simulink model "llc_ctrl_model"  (R2020a)
settings: Solver=ode45  StartTime=0.0  StopTime=1  RelTol=1e-3
undefined symbols (not defined in the file or in its folder): llc_ctrl_cfg_default
libraries: powerlib x19, commsynccomp2 x1
settings Model: Creator=huyan  LastModifiedBy=huyan

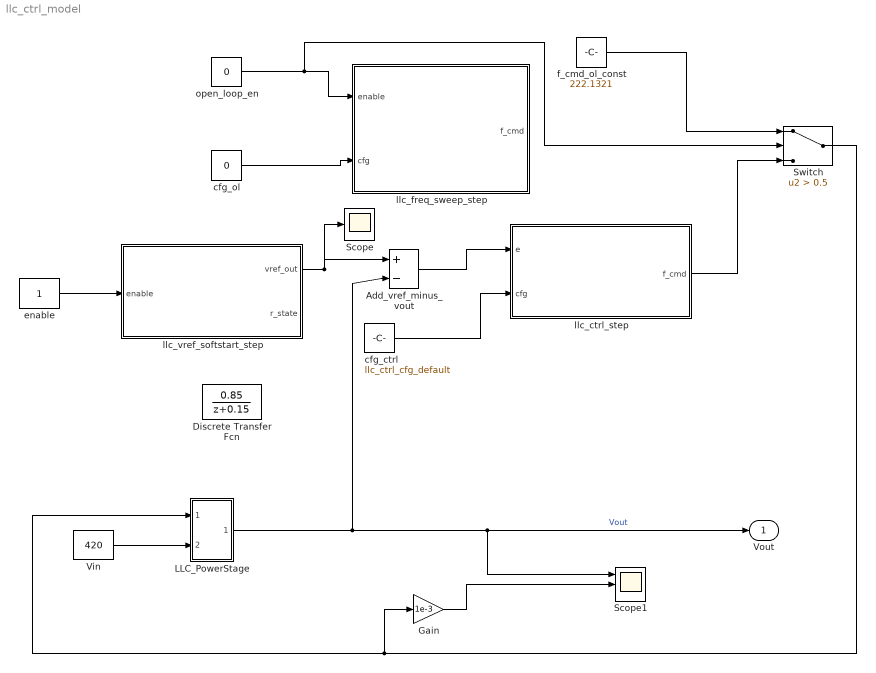
== system llc_ctrl_model ==
  Add_vref_minus_vout : Sum  Inputs=|+-
  Discrete Transfer Fcn : DiscreteTransferFcn  Numerator=0.85  Denominator=[1 0.15]  InitialStates=44  SampleTime=1e-4
  Gain : Gain  Gain=1e-3
  LLC_PowerStage : Subsystem
  Scope : Scope
  Scope1 : Scope  NumInputPorts=3
  Switch : Switch  Criteria=u2 > Threshold  Threshold=0.5
  Vin : Constant  Value=420  SampleTime=0.0001
  cfg_ctrl : Constant  Value=llc_ctrl_cfg_default  OutDataTypeStr=Bus: LLC_CTRL_CFG
  cfg_ol : Constant  Value=0  OutDataTypeStr=Bus: LLC_OL_CFG
  enable : Constant  SampleTime=0.0001
  f_cmd_ol_const : Constant  Value=222.1321
  llc_ctrl_step : MATLAB Function  TreatAsAtomicUnit=on  SystemSampleTime=1e-4
  "llc_freq_sweep_step " : MATLAB Function  TreatAsAtomicUnit=on
  llc_vref_softstart_step : MATLAB Function  TreatAsAtomicUnit=on  SystemSampleTime=1e-4
  open_loop_en : Constant  Value=0  OutDataTypeStr=double
  Vout : Outport
  wires:
  enable/1 -> llc_vref_softstart_step/1(enable)
  llc_vref_softstart_step/1(vref_out) -> Scope/1, Add_vref_minus_vout/1
  Add_vref_minus_vout/1 -> llc_ctrl_step/1(e)
  Vin/1 -> LLC_PowerStage/2(Vin)
  LLC_PowerStage/1(Vout) -> Add_vref_minus_vout/2, Vout/1, Scope1/1  "Vout"
  open_loop_en/1 -> "llc_freq_sweep_step "/1(enable), Switch/2
  cfg_ol/1 -> "llc_freq_sweep_step "/2(cfg)
  cfg_ctrl/1 -> llc_ctrl_step/2(cfg)
  Gain/1 -> Scope1/2
  f_cmd_ol_const/1 -> Switch/1
  llc_ctrl_step/1(f_cmd) -> Switch/3
  Switch/1 -> Gain/1, LLC_PowerStage/1(f_cmd)

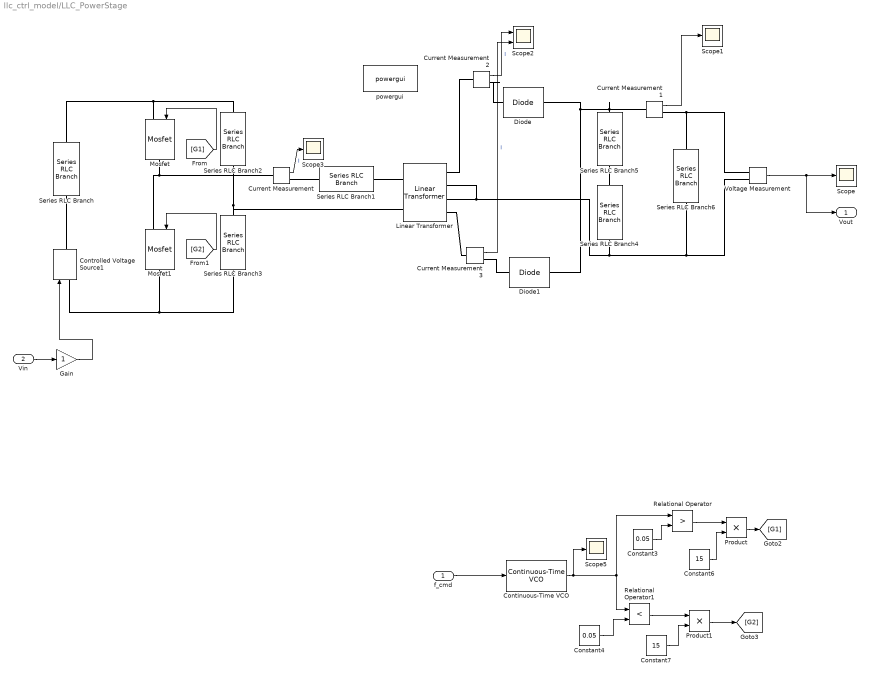
== system llc_ctrl_model/LLC_PowerStage ==
  f_cmd : Inport
  Vin : Inport  Port=2
  Constant3 : Constant  Value=0.05
  Constant4 : Constant  Value=0.05
  Constant6 : Constant  Value=15
  Constant7 : Constant  Value=15
  Continuous-Time VCO : commsynccomp2/Continuous-Time VCO  Ac=1  Fc=0  Kc=1  Ph=0
      settings: SourceProductBaseCode=CM
  Controlled Voltage Source1 : powerlib/Electrical Sources/Controlled Voltage Source  Initialize=on  Source_Type=AC  Amplitude=0  Phase=0  Frequency=0  Measurements=None
  Current Measurement{,1..3} (4 alike) : powerlib/Measurements/Current Measurement  PhasorSimulation=off  OutputType=Complex  PSBequivalent=0
  Diode : powerlib/Power Electronics/Diode  Ron=0.001  Lon=0  Vf=1.5  IC=0  UseSnubber=0  Rs=0.8  Cs=1e-9  Measurements=off
  Diode1 : powerlib/Power Electronics/Diode  Ron=0.001  Lon=0  Vf=1.5  IC=0  UseSnubber=0  Rs=0.8  Cs=1e-9  Measurements=off
  Gain : Gain
  Linear Transformer : powerlib/Elements/Linear Transformer  UNITS=SI  NominalPower=[ 3000 100000 ]  winding1=[300 0 0]  winding2=[63.1 0 0]  ThreeWindings=on  winding3=[63.1 0 0]  RmLm=[2.888e+08 0.000077]  Measurements=None  DataType=on
  Mosfet : powerlib/Power Electronics/Mosfet  Ron=0.1  Lon=0  Rd=0.01  Vfd=0  IC=0  Rs=1e5  Cs=inf  Measurements=off
  Mosfet1 : powerlib/Power Electronics/Mosfet  Ron=0.1  Lon=0  Rd=0.01  Vfd=0  IC=0  Rs=1e5  Cs=inf  Measurements=off
  Product : Product
  Product1 : Product
  Relational Operator : RelationalOperator  Operator=>  OutDataTypeStr=boolean  RndMeth=Simplest
  Relational Operator1 : RelationalOperator  Operator=<  OutDataTypeStr=boolean  RndMeth=Simplest
  Scope{,1,3,5} (4 alike) : Scope
  Scope2 : Scope  NumInputPorts=2
  Series RLC Branch : powerlib/Elements/Series RLC Branch  LConnTagsString=__new0  RConnTagsString=__new0  BranchType=R  Resistance=1E-3  Inductance=1e-3  SetiL0=off  InitialCurrent=0  Capacitance=1e-6  Setx0=off  InitialVoltage=0  Measurements=None
  Series RLC Branch1 : powerlib/Elements/Series RLC Branch  LConnTagsString=__new0  RConnTagsString=__new0  BranchType=L  Resistance=1E-3  Inductance=23e-6  SetiL0=off  InitialCurrent=0  Capacitance=1e-6  Setx0=off  InitialVoltage=0  Measurements=None
  Series RLC Branch2 : powerlib/Elements/Series RLC Branch  LConnTagsString=__new0  RConnTagsString=__new0  BranchType=C  Resistance=1E-3  Inductance=23e-3  SetiL0=off  InitialCurrent=0  Capacitance=66e-9  Setx0=off  InitialVoltage=0  Measurements=None
  Series RLC Branch3 : powerlib/Elements/Series RLC Branch  LConnTagsString=__new0  RConnTagsString=__new0  BranchType=C  Resistance=1E-3  Inductance=23e-3  SetiL0=off  InitialCurrent=0  Capacitance=66e-9  Setx0=off  InitialVoltage=0  Measurements=None
  Series RLC Branch4 : powerlib/Elements/Series RLC Branch  LConnTagsString=__new0  RConnTagsString=__new0  BranchType=C  Resistance=1E-3  Inductance=23e-3  SetiL0=off  InitialCurrent=0  Capacitance=12000e-6  Setx0=off  InitialVoltage=0  Measurements=None
  Series RLC Branch5 : powerlib/Elements/Series RLC Branch  LConnTagsString=__new0  RConnTagsString=__new0  BranchType=R  Resistance=0.015  Inductance=1e-3  SetiL0=off  InitialCurrent=0  Capacitance=1e-6  Setx0=off  InitialVoltage=0  Measurements=None
  Series RLC Branch6 : powerlib/Elements/Series RLC Branch  LConnTagsString=__new0  RConnTagsString=__new0  BranchType=R  Resistance=1.36875  Inductance=1e-3  SetiL0=off  InitialCurrent=0  Capacitance=1e-6  Setx0=off  InitialVoltage=0  Measurements=None
  Voltage Measurement : powerlib/Measurements/Voltage Measurement  PhasorSimulation=off  OutputType=Complex  PSBequivalent=0
  powergui : powerlib/powergui  Priority=1  SimulationMode=Discrete  SampleTime=1e-7  frequency=60  Iterations=50  frequencyindice=0  Pbase=100e6  ErrMax=1e-4  UnitsV=kV  UnitsW=MW  buscounter=0  FunctionMessages=off  echomessages=off  EnableUseOfTLC=off  CurrentSourceSwitches=off  DisableSnubberDevices=off  DisableRonSwitches=off  DisableVfSwitches=off  DisplayEquations=off  AutomaticDiscreteSolvers=off  SolverType=Tustin/Backward Euler (TBE)  Interpol=off  ExternalGateDelay=off  methode=off  Ts=100  x0status=blocks  SPID=on  SwTol=0  HookPort=off  NonlinearTolerance=1e-4  nMaxIteration=100  ContinueOnMaxIteration=off  RestoreLinks=warning  ResistiveCurrentMeasurement=off  Frange=[0:2:500]  Ylog=off  Xlog=on  ShowGrid=off  save=off  variable=ZData  structure=0  ZoomFFT=off  StartTime=0.0  cycles=1  DisplayStyle=1  fundamental=60  FreqAxis=off  MaxFrequency=1000  frequencyindicesteady=1  RmsSteady=1  display=off
  Vout : Outport
  wires:
  [G2] -> Mosfet1/1
  Current Measurement1/1 -> Scope1/1
  [G1] -> Mosfet/1
  Current Measurement/1 -> Scope3/1  "I"
  Vin/1 -> Gain/1
  Gain/1 -> Controlled Voltage Source1/1
  Voltage Measurement/1 -> Vout/1, Scope/1
  Product1/1 -> [G2]
  Constant4/1 -> Relational Operator1/2
  Product/1 -> [G1]
  Relational Operator1/1 -> Product1/1
  Relational Operator/1 -> Product/1
  Continuous-Time VCO/1 -> Scope5/1, Relational Operator/1, Relational Operator1/1
  Constant3/1 -> Relational Operator/2
  Constant6/1 -> Product/2
  Constant7/1 -> Product1/2
  f_cmd/1 -> Continuous-Time VCO/1
  Current Measurement2/1 -> Scope2/1  "I"
  Current Measurement3/1 -> Scope2/2  "I"
  connections:
  Series RLC Branch/LConn1 -- Mosfet/LConn1 -- Series RLC Branch2/LConn1
  Current Measurement/RConn1 -- Series RLC Branch1/RConn1
  Mosfet/RConn1 -- Mosfet1/LConn1 -- Current Measurement/LConn1
  Controlled Voltage Source1/RConn1 -- Series RLC Branch/RConn1
  Series RLC Branch6/RConn1 -- Voltage Measurement/LConn2 -- Series RLC Branch4/RConn1 -- Linear Transformer/RConn2 -- Linear Transformer/RConn3
  Series RLC Branch3/LConn1 -- Controlled Voltage Source1/LConn1 -- Mosfet1/RConn1
  Diode/RConn1 -- Series RLC Branch5/LConn1 -- Current Measurement1/LConn1 -- Diode1/RConn1
  Series RLC Branch2/RConn1 -- Linear Transformer/LConn2 -- Series RLC Branch3/RConn1
  Current Measurement1/RConn1 -- Voltage Measurement/LConn1 -- Series RLC Branch6/LConn1
  Series RLC Branch1/LConn1 -- Linear Transformer/LConn1
  Series RLC Branch5/RConn1 -- Series RLC Branch4/LConn1
  Linear Transformer/RConn1 -- Current Measurement2/LConn1
  Current Measurement2/RConn1 -- Diode/LConn1
  Linear Transformer/RConn4 -- Current Measurement3/LConn1
  Current Measurement3/RConn1 -- Diode1/LConn1

== matlab function llc_ctrl_model/llc_vref_softstart_step ==
  data: enable input; vref_out output; r_state output
function [vref_out, r_state] = llc_vref_softstart_step(enable)
%#codegen
% 最简单版 Vref 软启动：
% 输入:
%   enable   : 1 = 软启使能，0 = 关闭（清零）
% 输出:
%   vref_out : 当前参考电压 Vref (V)
%   r_state  : 0.0~1.0 的斜坡进度（可以不接线）

    % ---- persistent: 斜坡进度 0~1 ----
    persistent r
    if isempty(r)
        r = 0.0;
    end

    % ---- 固定参数（先写死，后面再做 cfg）----
    Ts          = 1e-4;   % 10 kHz 控制周期
    t_ramp      = 0.3;    % 0→目标电压，软启时间 0.3 s
    vref_target = 44.0;   % 目标输出电压 46 V

    if enable ~= 0
        % 软启 ON
        if t_ramp <= 0
            r = 1.0;
        else
            r = r + Ts / t_ramp;
            if r > 1.0
                r = 1.0;
            end
        end
    else
        % 软启 OFF
        r = 0.0;
    end

    vref_out = r * vref_target;
    r_state  = r;
end

== matlab function llc_ctrl_model/llc_freq_sweep_step  ==
  data: enable input; f_cmd output; cfg input
function f_cmd = llc_freq_sweep_step(enable, cfg)
%#codegen
% 开环扫频频率发生器（离散）
%
% 输入:
%   enable : 1=开始扫频，0=复位到起始频率
%   cfg    : Bus LLC_OL_CFG
%            - f_start   : 起始频率 (Hz)
%            - f_end     : 终止频率 (Hz)
%            - t_sweep_s : 扫频总时间 (s)
%            - Ts_s      : 采样周期 (s)
% 输出:
%   f_cmd  : 当前时刻输出的频率 (Hz)

    % 进度 0~1
    persistent r
    if isempty(r)
        r = 0.0;
    end

    Ts      = cfg.Ts_s;
    t_sweep = cfg.t_sweep_s;
    f_start = cfg.f_start;
    f_end   = cfg.f_end;

    if enable ~= 0
        % 扫频开启
        if t_sweep <= 0
            % 扫频时间非法，直接一步到终点
            r = 1.0;
        else
            r = r + Ts / t_sweep;
            if r > 1.0
                r = 1.0;    % 扫完就停在终点频率
            end
        end
    else
        % 未使能：复位到起点
        r = 0.0;
    end

    % 线性插值：r=0 → f_start，r=1 → f_end
    f_cmd = f_start + (f_end - f_start) * r;
end

== matlab function llc_ctrl_model/llc_ctrl_step ==
  data: e input; f_cmd output; cfg input
function f_cmd = llc_ctrl_step(e, cfg)
%#codegen
% LLC 电压环：离散 PI + 频率 / 斜率限幅 + 积分抗饱和
%
% 输入:
%   e   : 电压误差 (Vref - Vout)
%   cfg : 结构体，字段:
%         kp, ki, f_min, f_max, f_slew, alpha(可不用)
%
% 输出:
%   f_cmd : 目标频率 (Hz)

    % -------- persistent: 积分 & 上一拍频率 --------
    persistent integ f_prev
    if isempty(integ)
        integ = 0.0;
    end
    if isempty(f_prev)
        % 初始频率放在靠近工作点：比如 90~95 kHz
        f_prev = 90e3;
    end

    % -------- 读配置（带容错） --------
    kp     = cfg.kp;
    ki     = cfg.ki;
    f_min  = cfg.f_min;
    f_max  = cfg.f_max;
    f_slew = cfg.f_slew;

    % 容错：如果某些参数没设，用一个保底值
    if f_min <= 0 || f_min >= f_max
        f_min = 70e3;
    end
    if f_max <= f_min
        f_max = 150e3;
    end
    if f_slew <= 0
        f_slew = 1e3;    % 每步最多 1 kHz
    end
    if kp <= 0
        kp = 300;        % 保底 P
    end
    if ki <= 0
        ki = 2000;       % 保底 I（后面会按 Ts 折算）
    end

    % 这里假设控制环 Ts = 1/10k = 0.0001 s（你的模型现在就是 10 kHz）
    Ts = 1/10e3;
    ki_d = ki * Ts;      % 连续域 ki(1/s) → 离散积分增量

    % -------- 先算“未限幅”的 PI 输出 --------
    % 1) 更新积分（先不加抗饱和）
    integ_candidate = integ + ki_d * e;

    % 2) 线性控制量 u：认为 u = Δf （要从参考频率减多少）
    u = kp * e + integ_candidate;

    % 3) 目标频率（未限幅）
    %    这里选“从 f_nom - u”这种形式，让 e>0 时频率升高
    f_nom = 91e3;  % 名义工作点（可调），建议设到你想运行的 91 kHz
    f_req = f_nom + u;

    % -------- 频率限幅 + 积分抗饱和 --------
    f_sat = f_req;

    if f_sat > f_max
        f_sat = f_max;
    elseif f_sat < f_min
        f_sat = f_min;
    end

    % 抗饱和逻辑：
    % 如果频率已经在上限，且误差 e 仍然要求“再往上拉”（让 f 再增加），
    % 就暂时冻结积分；下限同理。
    freeze_I = false;
    if (f_sat >= f_max - 1 && e > 0)
        freeze_I = true;   % 上饱和且误差正，继续积分只会更顶
    elseif (f_sat <= f_min + 1 && e < 0)
        freeze_I = true;   % 下饱和且误差负
    end

    if freeze_I
        % 不更新 integ
    else
        % 更新并做积分限幅
        integ = integ_candidate;
        % 积分范围大概覆盖 (f_max - f_min)
        I_max =  (f_max - f_min);
        I_min = -(f_max - f_min);
        if integ > I_max
            integ = I_max;
        elseif integ < I_min
            integ = I_min;
        end
    end

    % -------- 斜率限幅 --------
    df = f_sat - f_prev;
    if df > f_slew
        f_cmd = f_prev + f_slew;
    elseif df < -f_slew
        f_cmd = f_prev - f_slew;
    else
        f_cmd = f_sat;
    end

    f_prev = f_cmd;
end
